simulink model "understandingof_int_deri_blocks"  (R2024b)
settings: Solver=VariableStepAuto  StartTime=0.0  StopTime=10.0  RelTol=1e-3
settings Model: Creator=admin  LastModifiedBy=admin

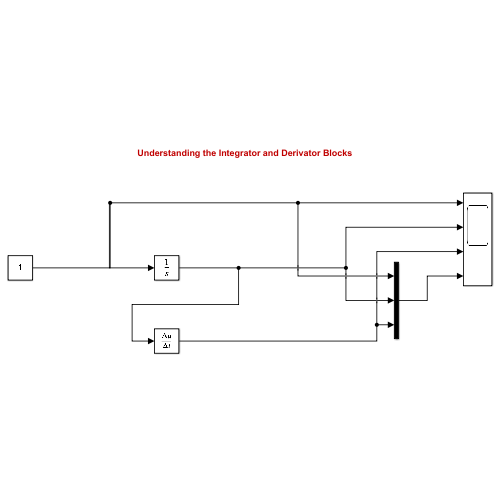
[thumbnail: Simulink's stored preview of the top-level diagram]
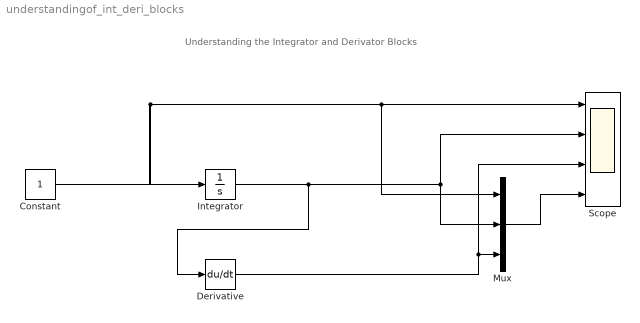
== system understandingof_int_deri_blocks ==
  note: Understanding the Integrator and Derivator Blocks
  Constant : Constant
  Derivative : Derivative
  Integrator : Integrator
  Mux : Mux  Inputs=3
  Scope : Scope  NumInputPorts=4
  wires:
  Constant/1 -> Mux/1, Scope/1, Integrator/1
  Integrator/1 -> Scope/2, Mux/2, Derivative/1
  Derivative/1 -> Scope/3, Mux/3
  Mux/1 -> Scope/4
